simulink model "valor_final_teorico"  (R2025a)
settings: Solver=VariableStepAuto  StartTime=0.0  StopTime=10.0  RelTol=1e-3
settings Model: Creator=dario  LastModifiedBy=dario

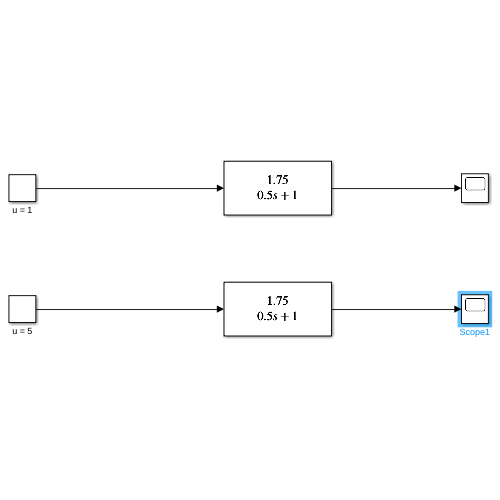
[thumbnail: Simulink's stored preview of the top-level diagram]
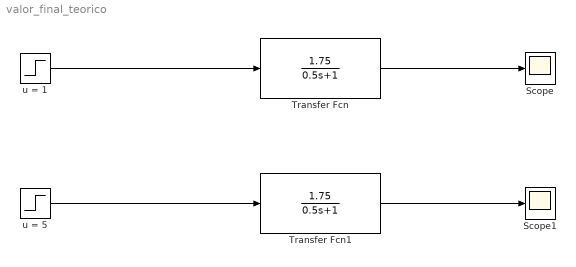
== system valor_final_teorico ==
  Scope : Scope
      settings: ActiveDisplayYMinimum=2.1064361121474722  ActiveDisplayYMaximum=11.336861315613735
  Scope1 : Scope
      settings: ActiveDisplayYMinimum=2.1064361121474722  ActiveDisplayYMaximum=11.336861315613735
  Transfer Fcn : TransferFcn  Numerator=[1.75]  Denominator=[0.5 1]
  Transfer Fcn1 : TransferFcn  Numerator=[1.75]  Denominator=[0.5 1]
  u = 1 : Step  SampleTime=0
  u = 5 : Step  After=5  SampleTime=0
  wires:
  Transfer Fcn/1 -> Scope/1
  u = 1/1 -> Transfer Fcn/1
  u = 5/1 -> Transfer Fcn1/1
  Transfer Fcn1/1 -> Scope1/1
